simulink model "program_nova_torque_vectoring_001_2015b"  (R2016a)
settings: Solver=FixedStepAuto  StartTime=0.0  StopTime=10.0  RelTol=1e-3
PreLoadFcn:
  | dataCar
  | load_vars
  | readFuzzyFile
  | structAero
  | structEstimPar
  | structSensors
  | structSettings
PostLoadFcn:
  | , if any(exist('dsrtsu_mdlpostloadfcn', 'file') == [2, 3, 6]), try dsrtsu_mdlpostloadfcn('Execute', bdroot); catch fprintf('Error in PostLoadFcn (dsrtsu_mdlpostloadfcn) for model "%s":\n %s\n', bdroot, lasterr); end, end,
InitFcn:
  | dataCar
  | load_vars
  | readFuzzyFile
  | structAero
  | structEstimPar
  | structSensors
  | structSettings
StartFcn:
  | dataCar
  | load_vars
  | readFuzzyFile
  | structAero
  | structEstimPar
  | structSensors
  | structSettings
values from neighbouring files (symbols this model uses):
  Throttle2_offset = 500    [load_vars.m]
  Throttle_limits = [0.15, 0.90, 0.16, 0.92]    [load_vars.m]
libraries: rtican x42, hdlsllib x32, simulink x3, fuzblock x1
(part 1 of 11)
settings Model: DSRTSU_INTERNAL_RTI_VER=490  DSRTSU_INTERNAL_RTI_TYPE=rti1401  DSRTSU_INTERNAL_RTIFPGA=80  Creator=Formula Electric  LastModifiedBy=Arthur Coppieters
settings DataIOCC: LimitDataPoints=on
settings DebuggingCC: AllowSymbolicDim=off
settings ModelReferenceCC: PropagateSignalLabelsOutOfModel=off
settings GRTTargetCC: GeneratePreprocessorConditionals=Use local settings
settings ConfigComp: CovModelRefEnable=Off
settings ConfigurationSet: Description=SimMechanics 2G

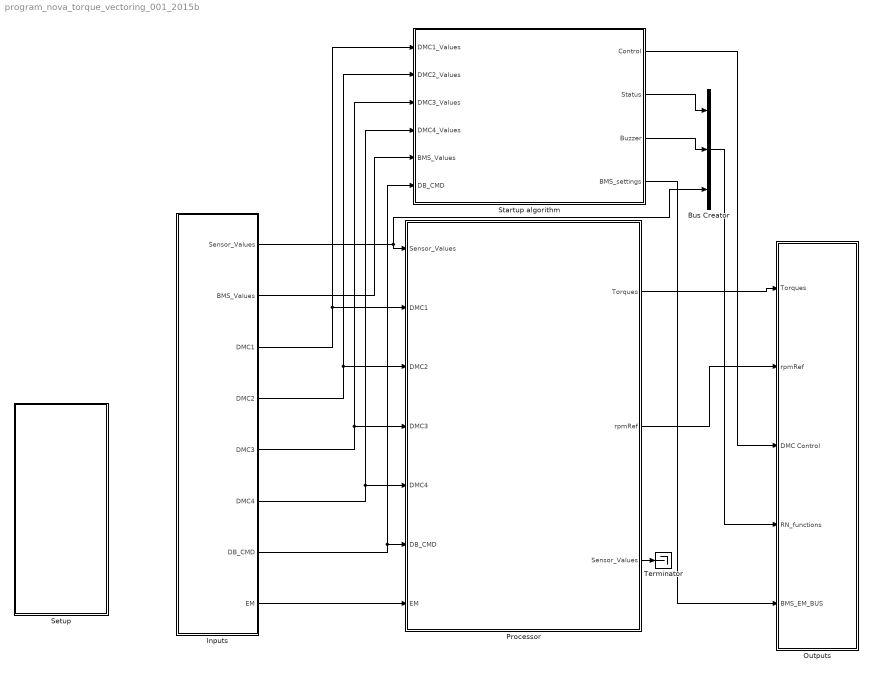
== system program_nova_torque_vectoring_001_2015b ==
  Bus Creator : BusCreator  Inputs=3
  Inputs : Subsystem
  Outputs : Subsystem
  Processor : Subsystem
  Setup : Subsystem
  Startup algorithm : Subsystem
  Terminator : Terminator
  wires:
  Inputs/1(Sensor_Values) -> Bus Creator/3, Processor/1("Sensor_Values ")
  Inputs/2(BMS_Values) -> Startup algorithm/5(BMS_Values)
  Inputs/3(DMC1) -> Startup algorithm/1(DMC1_Values), Processor/2(DMC1)
  Inputs/4(DMC2) -> Startup algorithm/2(DMC2_Values), Processor/3(DMC2)
  Inputs/5(DMC3) -> Startup algorithm/3(DMC3_Values), Processor/4(DMC3)
  Inputs/6(DMC4) -> Startup algorithm/4(DMC4_Values), Processor/5(DMC4)
  Inputs/7(DB_CMD) -> Startup algorithm/6(DB_CMD), Processor/6(DB_CMD)
  Processor/1(Torques) -> Outputs/1(Torques)
  Processor/2(rpmRef) -> Outputs/2(rpmRef)
  Inputs/8(EM) -> Processor/7(EM)
  Startup algorithm/1(Control) -> Outputs/3(DMC Control)
  Startup algorithm/3(Buzzer) -> Bus Creator/2
  Startup algorithm/2(Status) -> Bus Creator/1
  Bus Creator/1 -> Outputs/4(RN_functions)
  Startup algorithm/4(BMS_settings) -> Outputs/5(BMS_EM_BUS)
  Processor/3(Sensor_Values) -> Terminator/1

== system program_nova_torque_vectoring_001_2015b/Inputs ==
  Batpack : Subsystem
  Bus Creator : BusCreator  Inputs=4
  Commands : Subsystem
  Drives : Subsystem
  EnergyMeter : Subsystem
  Preprocessor : Subsystem
  Sensors : Subsystem
  Sensor_Values : Outport
  BMS_Values : Outport  Port=2
  DMC1 : Outport  Port=3
  DMC2 : Outport  Port=4
  DMC3 : Outport  Port=5
  DMC4 : Outport  Port=6
  DB_CMD : Outport  Port=7
  EM : Outport  Port=8
  wires:
  Batpack/1(BMS_Values) -> BMS_Values/1
  Drives/1(DMC1) -> DMC1/1
  Drives/2(DMC2) -> DMC2/1
  Drives/3(DMC3) -> DMC3/1
  Drives/4(DMC4) -> DMC4/1
  Commands/1(Dash_Commands) -> DB_CMD/1
  Sensors/1(Front_Sensors) -> Preprocessor/1(Front)
  Sensors/4(Temp_Sensors_Rear) -> Bus Creator/4
  Bus Creator/1 -> Sensor_Values/1  "Sensor_Values"
  Preprocessor/1(Front_proc) -> Bus Creator/1  "Front_proc"
  Sensors/2(Rear_Sensors) -> Preprocessor/2(Rear)
  Preprocessor/2(YRS) -> Bus Creator/2
  Sensors/3(Temp_Sensors_Front) -> Bus Creator/3
  EnergyMeter/1("EM ") -> EM/1

== system program_nova_torque_vectoring_001_2015b/Outputs ==
  Torques : Inport
  rpmRef : Inport  Port=2
  DMC Control : Inport  Port=3
  RN_functions : Inport  Port=4
  BMS_EM_BUS : Inport  Port=5
  BMS_EM : Subsystem
  Bus Creator{,1..3} (4 alike) : BusCreator  Inputs=4
  Bus Selector : BusSelector  OutputSignals=Status
  Dashboard : Subsystem
  Drives : Subsystem
  MATLAB Function : MATLAB Function  TreatAsAtomicUnit=on
  Rear Node : Subsystem
  wires:
  Bus Creator/1 -> Drives/1(DMC1)
  Bus Creator1/1 -> Drives/2(DMC2)
  Bus Creator2/1 -> Drives/3(DMC3)
  Bus Creator3/1 -> Drives/4(DMC4)
  Torques/1 -> MATLAB Function/1(Torques)
  MATLAB Function/1(torqueFL_Pos) -> Bus Creator/2
  MATLAB Function/2(torqueFL_Neg) -> Bus Creator/3
  MATLAB Function/4(torqueFR_Pos) -> Bus Creator1/2
  MATLAB Function/5(torqueFR_Neg) -> Bus Creator1/3
  MATLAB Function/7(torqueRL_Pos) -> Bus Creator2/2
  MATLAB Function/8(torqueRL_Neg) -> Bus Creator2/3
  MATLAB Function/10(torqueRR_Pos) -> Bus Creator3/2
  MATLAB Function/11(torqueRR_Neg) -> Bus Creator3/3
  MATLAB Function/3(wheelspeedFL) -> Bus Creator/1
  MATLAB Function/6(wheelspeedFR) -> Bus Creator1/1
  MATLAB Function/9(wheelspeedRL) -> Bus Creator2/1
  MATLAB Function/12(wheelspeedRR) -> Bus Creator3/1
  BMS_EM_BUS/1 -> BMS_EM/1(In1)
  DMC Control/1 -> Bus Creator3/4, Bus Creator2/4, Bus Creator1/4, Bus Creator/4  "ControlValue"
  RN_functions/1 -> Bus Selector/1, Rear Node/1(RN_CTRL)
  Bus Selector/1 -> MATLAB Function/2(status)  "<Status>"

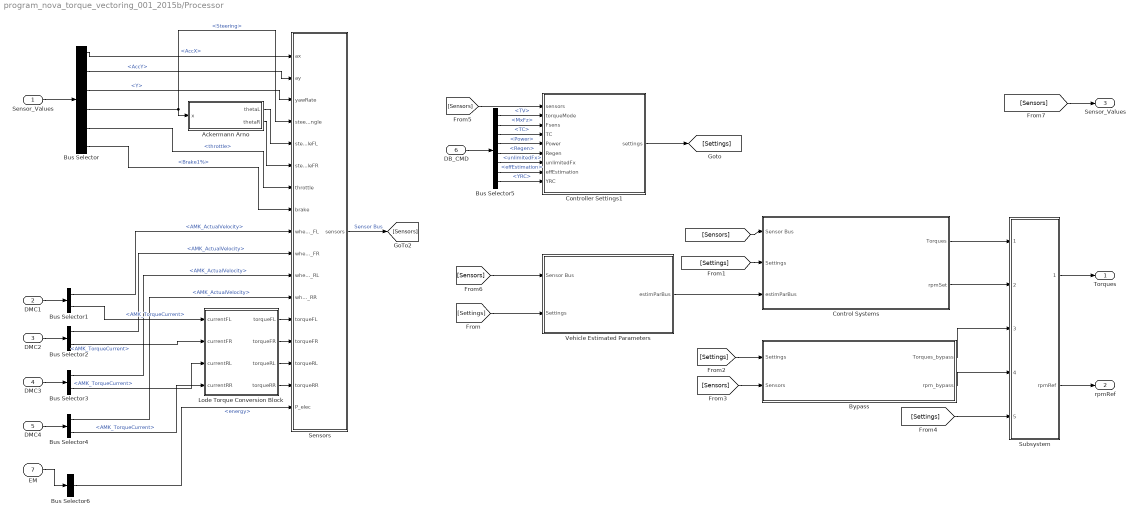
== system program_nova_torque_vectoring_001_2015b/Processor ==
  "Sensor_Values " : Inport
  DMC1 : Inport  Port=2
  DMC2 : Inport  Port=3
  DMC3 : Inport  Port=4
  DMC4 : Inport  Port=5
  DB_CMD : Inport  Port=6
  EM : Inport  Port=7
  Ackermann Arno : MATLAB Function  TreatAsAtomicUnit=on
  Bus Selector : BusSelector  OutputSignals=signal2.AccX,signal2.AccY,signal2.Y,Front_proc.Steering,Front_proc.throttle,Front_proc.Brake1%
  Bus Selector{1..4} (4 alike) : BusSelector  OutputSignals=AMK_ActualVelocity,AMK_TorqueCurrent
  Bus Selector5 : BusSelector  OutputSignals=TV,MxFz,TC,Power,Regen,unlimitedFx,effEstimation,YRC
  Bus Selector6 : BusSelector  OutputSignals=energy
  Bypass : Subsystem
  Control Systems : Subsystem
  Controller Settings1 : MATLAB Function  TreatAsAtomicUnit=on
  Lode Torque Conversion Block : MATLAB Function  TreatAsAtomicUnit=on
  Sensors : MATLAB Function  TreatAsAtomicUnit=on
  Subsystem : Subsystem
  Vehicle Estimated Parameters : Subsystem
  Torques : Outport
  rpmRef : Outport  Port=2
  Sensor_Values : Outport  Port=3
  wires:
  [Settings] -> Vehicle Estimated Parameters/2(Settings)
  Vehicle Estimated Parameters/1(" estimParBus") -> Control Systems/3(estimParBus)
  Controller Settings1/1(settings) -> [Settings]
  [Settings] -> Control Systems/2(Settings)
  Control Systems/1(Torques) -> Subsystem/1(TorqueController)
  Subsystem/1(Torques) -> Torques/1
  [Settings] -> Subsystem/5(Settings)
  Control Systems/2(rpmSet) -> Subsystem/2(rpmController)
  DB_CMD/1 -> Bus Selector5/1
  Subsystem/2(rpmRef) -> rpmRef/1
  [Sensors] -> Vehicle Estimated Parameters/1(Sensor Bus)
  [Sensors] -> Control Systems/1(Sensor Bus)
  [Sensors] -> Sensor_Values/1
  [Sensors] -> Controller Settings1/1(sensors)
  Bus Selector5/8 -> Controller Settings1/9(YRC)  "<YRC>"
  Bus Selector5/7 -> Controller Settings1/8(effEstimation)  "<effEstimation>"
  Bus Selector5/6 -> Controller Settings1/7(unlimitedFx)  "<unlimitedFx>"
  Bus Selector5/5 -> Controller Settings1/6(Regen)  "<Regen>"
  Bus Selector5/4 -> Controller Settings1/5(Power)  "<Power>"
  Bus Selector5/3 -> Controller Settings1/4(TC)  "<TC>"
  Bus Selector5/2 -> Controller Settings1/3(Fsens)  "<MxFz>"
  Bus Selector5/1 -> Controller Settings1/2(torqueMode)  "<TV>"
  Bypass/1(Torques_bypass) -> Subsystem/3(TorqueBypass)
  Bypass/2(rpm_bypass) -> Subsystem/4(rpmBypass)
  [Sensors] -> Bypass/2(Sensors)
  [Settings] -> Bypass/1(Settings)
  "Sensor_Values "/1 -> Bus Selector/1
  DMC1/1 -> Bus Selector1/1
  DMC2/1 -> Bus Selector2/1
  DMC3/1 -> Bus Selector3/1
  DMC4/1 -> Bus Selector4/1
  Bus Selector/4 -> Sensors/4(steeringAngle), Ackermann Arno/1(x)  "<Steering>"
  Bus Selector/5 -> Sensors/7(throttle)  "<throttle>"
  Bus Selector/6 -> Sensors/8(brake)  "<Brake1%>"
  Bus Selector/3 -> Sensors/3(yawRate)  "<Y>"
  Bus Selector/2 -> Sensors/2(ay)  "<AccY>"
  Bus Selector/1 -> Sensors/1(ax)  "<AccX>"
  Bus Selector1/1 -> Sensors/9(wheelspeed_FL)  "<AMK_ActualVelocity>"
  Bus Selector1/2 -> Lode Torque Conversion Block/1(currentFL)  "<AMK_TorqueCurrent>"
  Bus Selector2/1 -> Sensors/10(wheelspeed_FR)  "<AMK_ActualVelocity>"
  Bus Selector2/2 -> Lode Torque Conversion Block/2(currentFR)  "<AMK_TorqueCurrent>"
  Bus Selector3/1 -> Sensors/11(wheelspeed_RL)  "<AMK_ActualVelocity>"
  Bus Selector3/2 -> Lode Torque Conversion Block/3(currentRL)  "<AMK_TorqueCurrent>"
  Bus Selector4/1 -> Sensors/12(wheelspeed_RR)  "<AMK_ActualVelocity>"
  Bus Selector4/2 -> Lode Torque Conversion Block/4(currentRR)  "<AMK_TorqueCurrent>"
  Ackermann Arno/1(thetaL) -> Sensors/5(steerAngleFL)
  Ackermann Arno/2(thetaR) -> Sensors/6(steerAngleFR)
  Sensors/1(sensors) -> [Sensors]  "Sensor Bus"
  EM/1 -> Bus Selector6/1
  Bus Selector6/1 -> Sensors/17(P_elec)  "<energy>"
  Lode Torque Conversion Block/4(torqueRR) -> Sensors/16(torqueRR)
  Lode Torque Conversion Block/1(torqueFL) -> Sensors/13(torqueFL)
  Lode Torque Conversion Block/2(torqueFR) -> Sensors/14(torqueFR)
  Lode Torque Conversion Block/3(torqueRL) -> Sensors/15(torqueRL)
